simulink model "SolarInverter_DigitalTwin"  (R2019b)
settings: Solver=ode23tb  StartTime=0.0  StopTime=inf  RelTol=1e-3
InitFcn:
  | SolarInverter_Params();
values from neighbouring files (symbols this model uses):
  Fnom = 60    [SolarInverter_Params.m]
  Pnom = 112e3    (= 112000)    [SolarInverter_Params.m]
  reec_dbd1 = -0.1    [SolarInverter_Params.m]
  reec_dbd2 = 0.1    [SolarInverter_Params.m]
  reec_dPmax = 0.1    [SolarInverter_Params.m]
  reec_dPmin = -0.1    [SolarInverter_Params.m]
  reec_Imax = 1    [SolarInverter_Params.m]
  reec_Iqhl = 1.0    (= 1)    [SolarInverter_Params.m]
  reec_Iqll = -0.4    [SolarInverter_Params.m]
  reec_Kqi = 0.0    (= 0)    [SolarInverter_Params.m]
  reec_Kqp = 0    [SolarInverter_Params.m]
  reec_Kvi = 0.0    (= 0)    [SolarInverter_Params.m]
  reec_Kvp = 0.1    [SolarInverter_Params.m]
  reec_Pmax = 1.0    (= 1)    [SolarInverter_Params.m]
  reec_Pmin = 0    [SolarInverter_Params.m]
  reec_Qmax = 0.435    [SolarInverter_Params.m]
  reec_Qmin = -0.435    [SolarInverter_Params.m]
  reec_Tiq = 0.02    [SolarInverter_Params.m]
  reec_Tp = 0.02    [SolarInverter_Params.m]
  reec_Tpord = 0.1    [SolarInverter_Params.m]
  reec_Trv = 0.01    [SolarInverter_Params.m]
  reec_Vdip = 0.9    [SolarInverter_Params.m]
  reec_Vmax = 1.10    (= 1.1)    [SolarInverter_Params.m]
  reec_Vmin = 0.9    [SolarInverter_Params.m]
  reec_Vup = 1.15    [SolarInverter_Params.m]
  regc_Brkpt = 0.9    [SolarInverter_Params.m]
  regc_Iolim = -1.2    [SolarInverter_Params.m]
  regc_Iqrmax = 999.9    [SolarInverter_Params.m]
  regc_Iqrmin = -999.9    [SolarInverter_Params.m]
  regc_Ivpnt0 = 0.4    [SolarInverter_Params.m]
  regc_Ivpnt1 = 0.8    [SolarInverter_Params.m]
  regc_Khv = 0.0    (= 0)    [SolarInverter_Params.m]
  regc_Lvpl1 = 1.0    (= 1)    [SolarInverter_Params.m]
  regc_Lvplsw = 0    [SolarInverter_Params.m]
  regc_rrpwr = 10    [SolarInverter_Params.m]
  regc_Tfltr = 0.02    [SolarInverter_Params.m]
  regc_Tg = 0.1    [SolarInverter_Params.m]
  regc_Volim = 1.1    [SolarInverter_Params.m]
  regc_Zerox = 0.5    [SolarInverter_Params.m]
  repc_db1 = 0    [SolarInverter_Params.m]
  repc_Ddn = 20    [SolarInverter_Params.m]
  repc_Dup = 0    [SolarInverter_Params.m]
  repc_emax = 999    [SolarInverter_Params.m]
  repc_emin = -999    [SolarInverter_Params.m]
  repc_fdbd1 = 0.01*0    (= 0)    [SolarInverter_Params.m]
  repc_fdbd2 = -0.01*0    (= 0)    [SolarInverter_Params.m]
  repc_femax = 999    [SolarInverter_Params.m]
  repc_femin = -999    [SolarInverter_Params.m]
  repc_Kc = 0.05    [SolarInverter_Params.m]
  repc_Ki = 1.8    [SolarInverter_Params.m]
  repc_Kig = 0.5    [SolarInverter_Params.m]
  repc_Kp = 0.6    [SolarInverter_Params.m]
  repc_Kpg = 0.1    [SolarInverter_Params.m]
  repc_Pmax = 1    [SolarInverter_Params.m]
  repc_Pmin = 0    [SolarInverter_Params.m]
  repc_Qmax = inf    [SolarInverter_Params.m]
  repc_Qmin = -inf    [SolarInverter_Params.m]
  repc_Rc = 0    [SolarInverter_Params.m]
  repc_Tfltr = 0.02    [SolarInverter_Params.m]
  repc_Tft = 0.5    [SolarInverter_Params.m]
  repc_Tfv = 0.8    [SolarInverter_Params.m]
  repc_Tlag = 0.2    [SolarInverter_Params.m]
  repc_Tp = 0.25    [SolarInverter_Params.m]
  repc_Vfrz = 0.7    [SolarInverter_Params.m]
  repc_Xc = 0    [SolarInverter_Params.m]
  Vnom = 142e3    (= 142000)    [SolarInverter_Params.m]
undefined symbols (not defined in the file or in its folder): gcbh, j, sps_rtmsupport
libraries: simulink x15, powerlib x7, powerlib_meascontrol x2
(part 1 of 2)
settings Model: EnablePacing=on  OrderedModelArguments=off  Creator=jlesage  LastModifiedBy=jlesage
settings SolverCC: ZeroCrossAlgorithm=Adaptive
settings DataIOCC: InitialState=getstatestruct(opreport)  SaveOutput=off  SignalLogging=off  DSMLogging=off  SaveTime=off  ReturnWorkspaceOutputs=off
settings DebuggingCC: IgnoredZcDiagnostic=none
settings SFSimCC: CustomCodeUndefinedFunction=UseInterfaceOnly

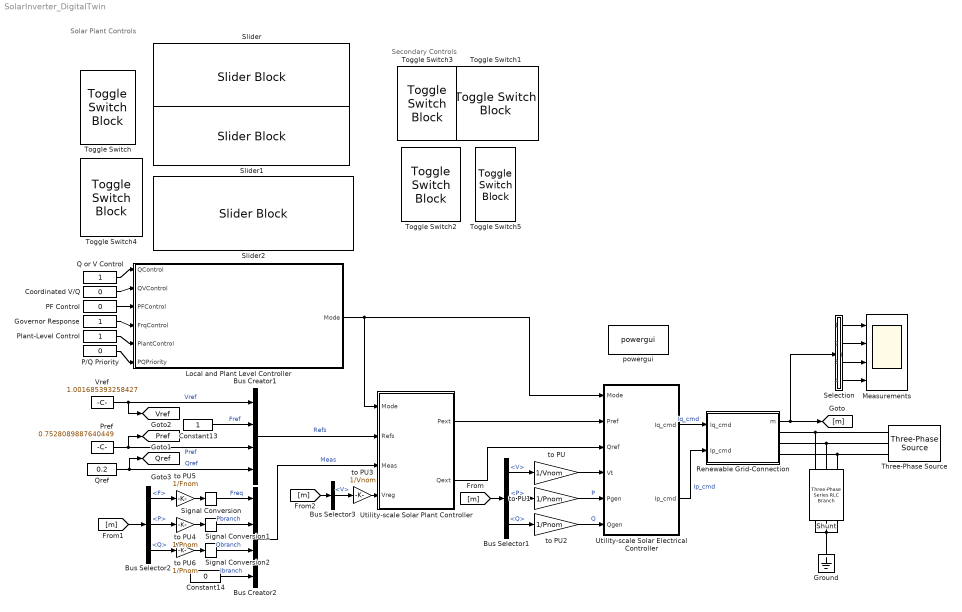
== system SolarInverter_DigitalTwin ==
  note: Solar Plant Controls
  note: Secondary Controls
  Bus Creator1 : BusCreator  Inputs=4
  Bus Creator2 : BusCreator  Inputs=4
  Bus Selector1 : BusSelector  OutputSignals=V,P,Q
  Bus Selector2 : BusSelector  OutputSignals=F,P,Q
  Bus Selector3 : BusSelector  OutputSignals=V
  Constant13 : Constant
  Constant14 : Constant  Value=0
  Coordinated V/Q : Constant  Value=0
  Governor Response : Constant
  Ground : powerlib/Elements/Ground  LConnTagsString=a
      settings: SourceProductName=Simscape Electrical
  Local and Plant Level Controller : Stateflow chart  InitFcn=|  BlockKeywords=__PRM__SERIALIZED__DATA__:Stateflow Chart,Stateflow Diagram  TreatAsAtomicUnit=on
      | BusElement(1) = Simulink.BusElement;
      | BusElement(1).Name = 'QFlag';
      | BusElement(1).Dimensions = 1;
      | BusElement(1).DimensionsMode = 'Fixed';
      | BusElement(1).DataType = 'double';
      | BusElement(1).Complexity = 'real';
      | 
      | BusElement(2) = Simulink.BusElement;
      | BusElement(2).Name = 'VFlag';
      | BusElement(2).Dimensions = 1;
      | BusElement(2).DimensionsMode = 'Fixed';
      | BusElement(2).DataType = 'double';
      | BusElement(2).Complexity = 'real';
      | 
      | BusElement(3) = Simulink.BusElement;
      | BusElement(3).Name = 'PfFlag';
      | BusElement(3).Dimensions = 1;
      | BusElement(3).DimensionsMode = 'Fixed';
      | BusElement(3).DataType = 'double';
      | BusElement(3).Complexity = 'real';
      | 
      | BusElement(4) = Simulink.BusElement;
      | BusElement(4).Name = 'PqFlag';
      | BusElement(4).Dimensions = 1;
      | BusElement(4).DimensionsMode = 'Fixed';
      | BusElement(4).DataType = 'double';
      | BusElement(4).Complexity = 'real';
      | 
      | BusElement(5) = Simulink.BusElement;
      | BusElement(5).Name = 'VcompFlag';
      | BusElement(5).Dimensions = 1;
      | BusElement(5).DimensionsMode = 'Fixed';
      | BusElement(5).DataType = 'double';
      | BusElement(5).Complexity = 'real';
      | 
      | BusElement(6) = Simulink.BusElement;
      | BusElement(6).Name = 'RefFlag';
      | BusElement(6).Dimensions = 1;
      | BusElement(6).DimensionsMode = 'Fixed';
      | BusElement(6).DataType = 'double';
      | BusElement(6).Complexity = 'real';
      | 
      | BusElement(7) = Simulink.BusElement;
      | BusElement(7).Name = 'FrqFlag';
      | BusElement(7).Dimensions = 1;
      | BusElement(7).DimensionsMode = 'Fixed';
      | BusElement(7).DataType = 'double';
      | BusElement(7).Complexity = 'real';
      | 
      | Mode = Simulink.Bus;
      | Mode.Elements = BusElement;
      | 
      | clearvars BusElement
  Measurements : Scope  NumInputPorts=4
  P/Q Priority : Constant  Value=0
  PF Control : Constant  Value=0
  Plant-Level Control : Constant
  Pref : Constant  Value=0.7528089887640449
  Q or V Control : Constant
  Qref : Constant  Value=0.2
  Renewable Grid-Connection : Subsystem  mask(Renewable Energy Grid Connection (REGC_A)){Tfltr=regc_Tfltr, Lvpl1=regc_Lvpl1, Zerox=regc_Zerox, Brkpt=regc_Brkpt, Lvplsw=regc_Lvplsw, rrpwr=regc_rrpwr, Tg=regc_Tg, Volim=regc_Volim, Iolim=regc_Iolim, Khv=regc_Khv, Ivpnt0=regc_Ivpnt0, Ivpnt1=regc_Ivpnt1, Iqrmax=regc_Iqrmax, Iqrmin=regc_Iqrmin}
      mask prompts: Tfltr "Tfltr - Terminal Voltage Filter [s]"; Lvpl1 "Lvpl1 - LVPL Gain Breakpoint [pu]"; Zerox "Zerox - LVPL Zero Crossing [pu]"; Brkpt "Brkpt - LVPL Breakpoint [pu]"; Lvplsw "Lvplsw - Low Voltage Power Logic [Enable (1) or Disable (0)]"; rrpwr "rrpwr - Active Current up-ramp rater limit [pu/s]"; Tg "Tg - Inverter Current Lag Time [s]"; Volim "Volim - Voltage Limit Clap Logic [pu]"; Iolim "Iolim - Current Limit for Clap Logic [pu]"; Khv "Khv - High Voltage Clap Logic Factor"; Ivpnt0 "Ivpnt0 - Low voltage current breakpoint [pu]"; Ivpnt1 "Ivpnt1 - Low voltage current breakpoint [pu]"; Iqrmax "Iqrmax - Maximum rate of change [pu/s]"; Iqrmin "Iqrmin - Minimum rate of change [pu/s]"
      mask help: REGC_A module, used to represent the Generator/Converter (inverter) interface with the grid. It processes the real and reactive current command and outputs of real and reactive current injection into the grid model.
      mask Display: color('blue');disp('REGC_A')
  Selection : Subsystem
  Shunt : powerlib/Elements/Three-Phase Series RLC Branch  LConnTagsString=A|B|C  RConnTagsString=A|B|C  BranchType=R  Resistance=1e9  Inductance=0  Capacitance=1e-6  Measurements=None
      settings: SourceProductName=Simscape Electrical
  Signal Conversion : SignalConversion  OverrideOpt=off
  Signal Conversion1 : SignalConversion  OverrideOpt=off
  Signal Conversion2 : SignalConversion  OverrideOpt=off
  Slider : SliderBlock  ScaleMin=0.94999999999999996  ScaleMax=1.05
  Slider1 : SliderBlock  ScaleMax=1  TickInterval=0.25
  Slider2 : SliderBlock  ScaleMin=-1  ScaleMax=1
  Three-Phase Source : powerlib/Electrical Sources/Three-Phase Source  InternalConnection=Yg  VoltagePhases=off  Voltage=Vnom*0.995  PhaseAngle=0  Voltage_phases=[25e3 25e3 25e3]/sqrt(3)  PhaseAngles_phases=[0 -120 +120]  Frequency=60  NonIdealSource=on  SpecifyImpedance=on  Resistance=0.8929  Inductance=16.58e-3  ShortCircuitLevel=20e5  BaseVoltage=Vnom  XRratio=10  BusType=swing  Pref=10e3  Qref=0  Prefabc=[10e3, 10e3, 10e3]  Qrefabc=[0, 0, 0]  Qmin=-inf  Qmax=inf
      settings: SourceProductName=Simscape Electrical
  Toggle Switch{,1..5} (6 alike) : ToggleSwitchBlock  LabelPosition=Hide
  Utility-scale Solar Electrical Controller : Subsystem  mask(Renewable Energy Electrical Controller (REEC_B)){Trv=reec_Trv, Vdip=reec_Vdip, Vup=reec_Vup, dbd1=reec_dbd1, dbd2=reec_dbd2, Kqv=0, Iqhl=reec_Iqhl, Iqll=reec_Iqll, Tp=reec_Tp, Qmax=reec_Qmax, Qmin=reec_Qmin, Kqp=reec_Kqp, Kqi=reec_Kqi, Vmax=reec_Vmax, Vmin=reec_Vmin, Kvp=reec_Kvp, Kvi=reec_Kvi, Tiq=reec_Tiq, Tpord=reec_Tpord, Pmax=reec_Pmax, Pmin=reec_Pmin, dPmax=reec_dPmax, dPmin=reec_dPmin, Imax=reec_Imax}
      mask prompts: Trv "Trv - Terminal Bus Filter [s]"; Vdip "Vdip - Low Voltage Trigger [pu]"; Vup "Vup - High Voltage Trigger [pu]"; dbd1 "dbd1 - Overvoltage deadband [pu]"; dbd2 "dbd2 - Undervoltage deadband [pu]"; Kqv "Kqv - Reactive current injection gain [pu]"; Iqhl "Iqhl - Maximum current injection [pu]"; Iqll "Iqll - Minimum current injection [pu]"; Tp "Tp - Active Power Time Constant [s]"; Qmax "Qmax - Maximum reactive power [pu]"; Qmin "Qmin - Minimum reactive power [pu]"; Kqp "Kqp - Local Q regulator [pu]"; Kqi "Kqi - Local Q integrator gain [pu]"; Vmax "Vmax - Maximum inverter voltage [pu]"; Vmin "Vmin - Minium inverter terminal voltage [pu]"; Kvp "Kvp - Voltage Regulator Gain [pu]"; Kvi "Kvi - Voltage Integrator Gain [pu]"; Tiq "Tiq - Reactive Power Lag [s]"; Tpord "Tpord - Inverter Lag Time Constant [s]"; Pmax "Pmax - Maximum active power [pu]"; Pmin "Pmin - Minimum active power [pu]"; dPmax "dPmax - Power Up-ramp Limit [pu/s]"; dPmin "dPmin - Power Down-ramp Limit [pu/s]"; Imax "Imax - Maximum apparent current [pu]"
      mask help: REEC_B module, used to represent the Electrical Controls of the inverters. It acts on the active and reactive power reference from the REPC_A module, with feedback of terminal voltage and generator power output, and provides real and reactive current commands to the REGC_A module.
      mask Display: color('blue');disp('REEC_A')
  Utility-scale Solar Plant Controller : Subsystem  mask(Renewable Energy Plant Controller (REPC_A)){Tfltr=repc_Tfltr, Xc=repc_Xc, Rc=repc_Rc, Kc=repc_Kc, db1=repc_db1, emax=repc_emax, emin=repc_emin, Kp=repc_Kp, Ki=repc_Ki, Qmax=repc_Qmax, Qmin=repc_Qmin, Vfrz=repc_Vfrz, Tft=repc_Tft, Tfv=repc_Tfv, fdbd1=repc_fdbd1, fdbd2=repc_fdbd2, Ddn=repc_Ddn, Dup=repc_Dup, Tp=repc_Tp, femax=repc_femax, femin=repc_femin, Kpg=repc_Kpg, Kig=repc_Kig, Tlag=repc_Tlag, Pmax=repc_Pmax, Pmin=repc_Pmin}
      mask prompts: Tfltr "Tfltr - Voltage/Reactive Power Time Constants [s]"; Xc "Xc - Line drop compensation reactance [pu]"; Rc "Rc - Line drop compensation resistance [pu]"; Kc "Kc - Reactive droop [pu]"; db1 "db - Reactive power deadline [pu]"; emax "emax - Maximum Volt/VAR error [pu]"; emin "emin - Minimum Volt/VAR error [pu]"; Kp "Kp - Volt/VAR Propotional Gain [pu/pu]"; Ki "Ki - Volt/VAR Integral Gain [pu/pu-s]"; Qmax "Qmax - Max Plant Reactive Power [pu]"; Qmin "Qmin - Min Plant Reactive Power [pu]"; Vfrz "Vfrz - Voltage for Freezing Volt/VAR Integrator [pu]"; Tft "Tft - Q Lead Time Constant [s]"; Tfv "Tfv - Q Lag Time Constant [s]"; fdbd1 "fdbd1 - Overfrequency deadband for govenor [pu]"; fdbd2 "fdbd2 - Underfrequency deadband for govenor [pu]"; Ddn "Ddn - Down regulation droop [pu]"; Dup "Dup - Up regulation droop [pu]"; Tp "Tp - Active Power Filter Time Constant [s]"; femax "femax - Maximum Power Error [pu]"; femin "femin - Minimum Power Error [pu]"; Kpg "Kpg - Droop regulator gain [pu]"; Kig "Kig - Droop integral gain [pu]"; Tlag "Tlag - Plant Controller P output Lag [s]"; Pmax "Pmax - Maximum Plant Active Power [pu]"; Pmin "Pmin - Minimum Plant Active Power [pu]"
      mask help: REPC_A module, used to represent the Plant Controller. It processes voltage and reactive power output to emulate volt/var control at the plant level. It also processes frequency and active power output to emulate active power control. This module provides active reactive power command to the REEC_B module.
      mask Display: color('blue');disp('REPC_A')
  Vref : Constant  Value=1.001685393258427
  powergui : powerlib/powergui  Priority=1  SimulationMode=Phasor  SampleTime=50e-6  frequency=60  Iterations=50  frequencyindice=60  Pbase=100e6  ErrMax=1e-4  UnitsV=kV  UnitsW=MW  buscounter=0  FunctionMessages=off  echomessages=off  EnableUseOfTLC=off  CurrentSourceSwitches=off  DisableSnubberDevices=off  DisableRonSwitches=off  DisableVfSwitches=off  DisplayEquations=off  AutomaticDiscreteSolvers=off  SolverType=Tustin/Backward Euler (TBE)  Interpol=off  ExternalGateDelay=off  methode=off  Ts=100  x0status=blocks  SPID=on  SwTol=0  HookPort=off  NonlinearTolerance=0  nMaxIteration=15  ContinueOnMaxIteration=off  RestoreLinks=warning  ResistiveCurrentMeasurement=off  Frange=[0:2:500]  Ylog=off  Xlog=on  ShowGrid=off  save=off  variable=ZData  structure=0  ZoomFFT=off  StartTime=0.0  cycles=1  DisplayStyle=1  fundamental=60  FreqAxis=off  MaxFrequency=1000  frequencyindicesteady=1  RmsSteady=1  display=off
      settings: SourceProductName=Simscape Electrical
  to PU : Gain  Gain=1/Vnom
  to PU{1..2,4,6} (4 alike) : Gain  Gain=1/Pnom
  to PU3 : Gain  Gain=1/Vnom
  to PU5 : Gain  Gain=1/Fnom
  tag scope: Pref=global, Qref=global, Vref=global
  wires:
  Renewable Grid-Connection/1(m) -> [m], Selection/1(In1)
  Utility-scale Solar Plant Controller/1(Pext) -> Utility-scale Solar Electrical Controller/2(Pref)
  Bus Selector1/3 -> to PU2/1  "<Q>"
  Bus Selector1/1 -> to PU/1  "<V>"
  Bus Selector1/2 -> to PU1/1  "<P>"
  [m] -> Bus Selector1/1
  to PU/1 -> Utility-scale Solar Electrical Controller/4(Vt)
  Utility-scale Solar Electrical Controller/1(Iq_cmd) -> Renewable Grid-Connection/1(Iq_cmd)  "Iq_cmd"
  Utility-scale Solar Electrical Controller/2(Ip_cmd) -> Renewable Grid-Connection/2(Ip_cmd)  "Ip_cmd"
  to PU1/1 -> Utility-scale Solar Electrical Controller/5(Pgen)  "P"
  to PU2/1 -> Utility-scale Solar Electrical Controller/6(Qgen)  "Q"
  Bus Selector2/3 -> to PU6/1  "<Q>"
  to PU6/1 -> Signal Conversion2/1
  Signal Conversion2/1 -> Bus Creator2/3  "Qbranch"
  Signal Conversion/1 -> Bus Creator2/1  "Freq"
  to PU3/1 -> Utility-scale Solar Plant Controller/4(Vreg)
  Bus Creator1/1 -> Utility-scale Solar Plant Controller/2(Refs)  "Refs"
  Signal Conversion1/1 -> Bus Creator2/2  "Pbranch"
  to PU5/1 -> Signal Conversion/1
  Constant13/1 -> Bus Creator1/2  "Fref"
  Bus Selector2/2 -> to PU4/1  "<P>"
  [m] -> Bus Selector3/1
  Pref/1 -> Bus Creator1/3, [Pref]  "Pref"
  Bus Creator2/1 -> Utility-scale Solar Plant Controller/3(" Meas")  "Meas"
  Constant14/1 -> Bus Creator2/4  "Ibranch"
  Bus Selector2/1 -> to PU5/1  "<F>"
  Qref/1 -> [Qref], Bus Creator1/4  "Qref"
  [m] -> Bus Selector2/1
  to PU4/1 -> Signal Conversion1/1
  Bus Selector3/1 -> to PU3/1  "<V>"
  Utility-scale Solar Plant Controller/2(Qext) -> Utility-scale Solar Electrical Controller/3(Qref)
  Vref/1 -> Bus Creator1/1, [Vref]  "Vref"
  Local and Plant Level Controller/1(Mode) -> Utility-scale Solar Plant Controller/1(Mode), Utility-scale Solar Electrical Controller/1(Mode)
  P/Q Priority/1 -> Local and Plant Level Controller/6(PQPriority)
  Plant-Level Control/1 -> Local and Plant Level Controller/5(PlantControl)
  Governor Response/1 -> Local and Plant Level Controller/4(FrqControl)
  PF Control/1 -> Local and Plant Level Controller/3(PFControl)
  Coordinated V/Q/1 -> Local and Plant Level Controller/2(QVControl)
  Q or V Control/1 -> Local and Plant Level Controller/1(QControl)
  Selection/1(Out1) -> Measurements/1
  Selection/2(<F>) -> Measurements/2
  Selection/3(Out3) -> Measurements/3
  Selection/4(Out4) -> Measurements/4
  connections:
  Shunt/LConn3 -- Three-Phase Source/RConn3 -- Renewable Grid-Connection/RConn3
  Shunt/LConn1 -- Three-Phase Source/RConn1 -- Renewable Grid-Connection/RConn1
  Shunt/RConn2 -- Ground/LConn1 -- Shunt/RConn3 -- Shunt/RConn1
  Shunt/LConn2 -- Three-Phase Source/RConn2 -- Renewable Grid-Connection/RConn2

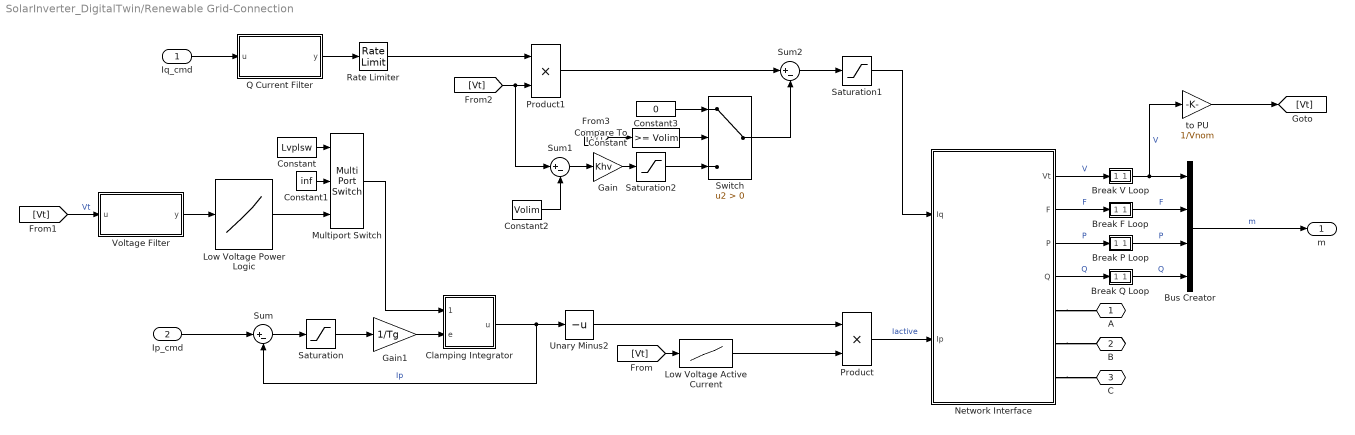
== system SolarInverter_DigitalTwin/Renewable Grid-Connection ==
  Iq_cmd : Inport
  Ip_cmd : Inport  Port=2
  Break F Loop : Subsystem  mask{tau=0.001, toPU=Fnom}
      mask prompts: toPU "Convert to PU"
  Break P Loop : Subsystem  mask{tau=0.001, toPU=Pnom}
      mask prompts: toPU "Convert to PU"
  Break Q Loop : Subsystem  mask{tau=0.001, toPU=Pnom}
      mask prompts: toPU "Convert to PU"
  Break V Loop : Subsystem  mask{tau=0.001, toPU=Vnom}
      mask prompts: toPU "Convert to PU"
  Bus Creator : BusCreator  Inputs=4
  Clamping Integrator : Subsystem
  Compare To Constant : simulink/Logic and Bit Operations/Compare To Constant  relop=>=  const=Volim  OutDataTypeStr=boolean
  Constant : Constant  Value=Lvplsw
  Constant1 : Constant  Value=inf
  Constant2 : Constant  Value=Volim
  Constant3 : Constant  Value=0
  Gain : Gain  Gain=Khv
  Gain1 : Gain  Gain=1/Tg
  Low Voltage Active Current : Lookup_n-D  NumberOfTableDimensions=1  BreakpointsForDimension1=[0 Ivpnt0 Ivpnt1 Ivpnt1*1.5]  Table=[0 0 1 1]  InternalRulePriority=Speed  RndMeth=Simplest  InputSameDT=on
  Low Voltage Power Logic : Lookup_n-D  NumberOfTableDimensions=1  BreakpointsForDimension1=[0 Zerox Brkpt Brkpt*1.01 Brkpt*1.5]  Table=[0 0 Lvpl1 Lvpl1*5 Lvpl1*5]  InternalRulePriority=Speed  RndMeth=Simplest  InputSameDT=on
  Multiport Switch : MultiPortSwitch  DataPortOrder=Zero-based contiguous  Inputs=2  zeroidx=on
  Network Interface : Subsystem
  Product : Product
  Product1 : Product
  Q Current Filter : Subsystem  mask{k=1, tau=Tg, vmax=Iqrmax, vmin=Iqrmin}
      mask Display: fprintf('1\n------------\n(1 + s Tg)');
  Rate Limiter : RateLimiter  RisingSlewLimit=Iqrmax  FallingSlewLimit=Iqrmin  SampleTimeMode=inherited
  Saturation : Saturate  UpperLimit=rrpwr  LowerLimit=-inf
  Saturation1 : Saturate  UpperLimit=inf  LowerLimit=Iolim
  Saturation2 : Saturate  UpperLimit=inf  LowerLimit=0
  Sum : Sum  Inputs=|+-
  Sum1 : Sum  Inputs=|+-
  Sum2 : Sum  Inputs=|+-
  Switch : Switch  Criteria=u2 > Threshold
  Unary Minus2 : UnaryMinus
  Voltage Filter : Subsystem  mask{k=1, tau=Tfltr, vmax=inf, vmin=-inf}
      mask Display: fprintf('1\n------------\n(1 + s Tfltr)');
  to PU : Gain  Gain=1/Vnom
  A : PMIOPort  Side=Right
  B : PMIOPort  Port=2  Side=Right
  C : PMIOPort  Port=3  Side=Right
  m : Outport  VectorParamsAs1DForOutWhenUnconnected=off
  wires:
  [Vt] -> Voltage Filter/1(u)  "Vt"
  Q Current Filter/1(y) -> Rate Limiter/1
  Network Interface/4(Q) -> Break Q Loop/1(u)  "Q"
  Constant3/1 -> Switch/1
  Network Interface/1(Vt) -> Break V Loop/1(u)  "V"
  Iq_cmd/1 -> Q Current Filter/1(u)
  Gain/1 -> Saturation2/1
  Network Interface/3(P) -> Break P Loop/1(u)  "P"
  Voltage Filter/1(y) -> Low Voltage Power Logic/1
  Constant1/1 -> Multiport Switch/2
  Sum/1 -> Saturation/1
  Constant/1 -> Multiport Switch/1
  Product/1 -> Network Interface/2(Ip)  "Iactive"
  Low Voltage Active Current/1 -> Product/2
  Multiport Switch/1 -> Clamping Integrator/1(LVMax)
  Clamping Integrator/1(u) -> Sum/2, Unary Minus2/1  "Ip"
  Gain1/1 -> Clamping Integrator/2(e)
  [Vt] -> Compare To Constant/1
  Saturation/1 -> Gain1/1
  [Vt] -> Low Voltage Active Current/1
  Constant2/1 -> Sum1/2
  Saturation1/1 -> Network Interface/1(Iq)
  Product1/1 -> Sum2/1
  Sum1/1 -> Gain/1
  Rate Limiter/1 -> Product1/1
  Saturation2/1 -> Switch/3
  [Vt] -> Sum1/1, Product1/2
  Low Voltage Power Logic/1 -> Multiport Switch/3
  Compare To Constant/1 -> Switch/2
  Switch/1 -> Sum2/2
  Bus Creator/1 -> m/1  "m"
  Sum2/1 -> Saturation1/1
  Ip_cmd/1 -> Sum/1
  Network Interface/2(F) -> Break F Loop/1(u)  "F"
  Unary Minus2/1 -> Product/1
  to PU/1 -> [Vt]
  Break V Loop/1(y) -> to PU/1, Bus Creator/1  "V"
  Break F Loop/1(y) -> Bus Creator/2  "F"
  Break P Loop/1(y) -> Bus Creator/3  "P"
  Break Q Loop/1(y) -> Bus Creator/4  "Q"
  connections:
  Network Interface/RConn3 -- C/RConn1
  Network Interface/RConn1 -- A/RConn1
  Network Interface/RConn2 -- B/RConn1

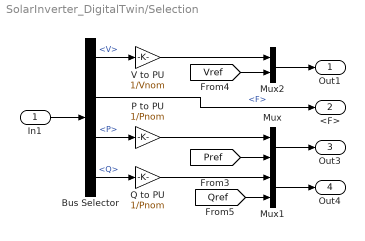
== system SolarInverter_DigitalTwin/Selection ==
  In1 : Inport
  Bus Selector : BusSelector  OutputSignals=V,F,P,Q
  Mux : Mux  Inputs=2
  Mux1 : Mux  Inputs=2
  Mux2 : Mux  Inputs=2
  P to PU : Gain  Gain=1/Pnom
  Q to PU : Gain  Gain=1/Pnom
  V to PU : Gain  Gain=1/Vnom
  Out1 : Outport
  <F> : Outport  Port=2
  Out3 : Outport  Port=3
  Out4 : Outport  Port=4
  wires:
  Bus Selector/4 -> Q to PU/1  "<Q>"
  Bus Selector/3 -> P to PU/1  "<P>"
  V to PU/1 -> Mux2/1
  Bus Selector/1 -> V to PU/1  "<V>"
  [Vref] -> Mux2/2
  Q to PU/1 -> Mux1/1
  P to PU/1 -> Mux/1
  [Qref] -> Mux1/2
  [Pref] -> Mux/2
  Bus Selector/2 -> <F>/1  "<F>"
  Mux/1 -> Out3/1
  Mux2/1 -> Out1/1
  Mux1/1 -> Out4/1
  In1/1 -> Bus Selector/1

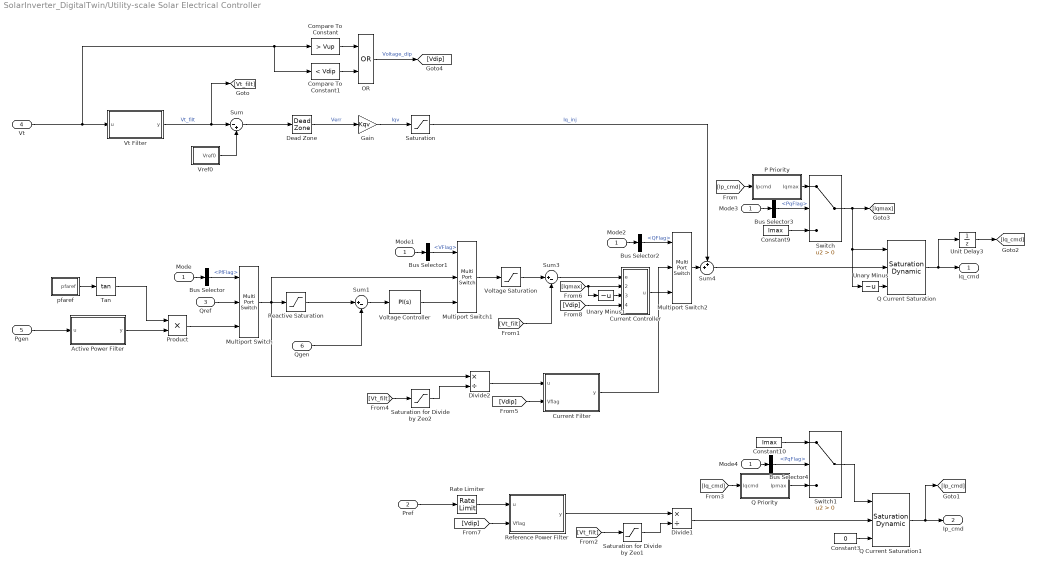
== system SolarInverter_DigitalTwin/Utility-scale Solar Electrical Controller ==
  Mode : Inport
  Pref : Inport  Port=2
  Qref : Inport  Port=3
  Vt : Inport  Port=4
  Pgen : Inport  Port=5
  Qgen : Inport  Port=6
  Active Power Filter : Subsystem  mask{k=1, tau=Tp, vmax=Inf, vmin=-Inf}
      mask Display: fprintf('1\n------------\n(1 + s Tp)');
  Bus Selector : BusSelector  OutputSignals=PfFlag
  Bus Selector1 : BusSelector  OutputSignals=VFlag
  Bus Selector2 : BusSelector  OutputSignals=QFlag
  Bus Selector3 : BusSelector  OutputSignals=PqFlag
  Bus Selector4 : BusSelector  OutputSignals=PqFlag
  Compare To Constant : simulink/Logic and Bit Operations/Compare To Constant  relop=>  const=Vup  OutDataTypeStr=boolean
  Compare To Constant1 : simulink/Logic and Bit Operations/Compare To Constant  relop=<  const=Vdip  OutDataTypeStr=boolean
  Constant10 : Constant  Value=Imax
  Constant3 : Constant  Value=0
  Constant9 : Constant  Value=Imax
  Current Controller : Subsystem
  Current Filter : Subsystem  mask{k=1, tau=Tiq, vmax=Inf, vmin=-Inf}
      mask Display: fprintf('1\n------------\n(1 + s Tiq)');
  Dead Zone : DeadZone  LowerValue=dbd1  UpperValue=dbd2  SaturateOnIntegerOverflow=on
  Divide1 : Product  Inputs=*/
  Divide2 : Product  Inputs=*/
  Gain : Gain  Gain=Kqv
  Mode{1..4} (4 alike) : InportShadow
  Multiport Switch : MultiPortSwitch  DataPortOrder=Zero-based contiguous  Inputs=2  zeroidx=on
  Multiport Switch1 : MultiPortSwitch  DataPortOrder=Zero-based contiguous  Inputs=2  zeroidx=on
  Multiport Switch2 : MultiPortSwitch  DataPortOrder=Zero-based contiguous  Inputs=2  zeroidx=on
  OR : Logic  Operator=OR  AllPortsSameDT=off  OutDataTypeStr=boolean
  P Priority : Subsystem
  Product : Product
  Q Current Saturation : simulink/Discontinuities/Saturation Dynamic  OutMin=[]  OutMax=[]  OutDataTypeStr=Inherit: Same as second input  OutDataType=fixdt(1, 16)  OutScaling=2^-10  DoSatur=off
  Q Current Saturation1 : simulink/Discontinuities/Saturation Dynamic  OutMin=[]  OutMax=[]  OutDataTypeStr=Inherit: Same as second input  OutDataType=fixdt(1, 16)  OutScaling=2^-10  DoSatur=off
  Q Priority : Subsystem
  Rate Limiter : RateLimiter  RisingSlewLimit=dPmax  FallingSlewLimit=dPmin  SampleTimeMode=inherited
  Reactive Saturation : Saturate  UpperLimit=Qmax  LowerLimit=Qmin
  Reference Power Filter : Subsystem  mask{k=1, tau=Tpord, vmax=Pmax, vmin=Pmin}
      mask Display: fprintf('1\n------------\n(1 + s Tpord)');
  Saturation : Saturate  UpperLimit=Iqhl  LowerLimit=Iqll
  Saturation for Divide by Zeo1 : Saturate  UpperLimit=inf  LowerLimit=0.01
  Saturation for Divide by Zeo2 : Saturate  UpperLimit=inf  LowerLimit=0.01
  Sum : Sum  Inputs=|-+
  Sum1 : Sum  Inputs=|+-
  Sum3 : Sum  Inputs=|+-
  Sum4 : Sum  Inputs=++|
  Switch : Switch  Criteria=u2 > Threshold
  Switch1 : Switch  Criteria=u2 > Threshold
  Tan : Trigonometry  Operator=tan
  Unary Minus : UnaryMinus
  Unary Minus1 : UnaryMinus
  Unit Delay3 : UnitDelay  SampleTime=-1  HasFrameUpgradeWarning=on
  Voltage Controller : simulink/Continuous/PID Controller  Controller=PI  Form=Parallel  TimeDomain=Continuous-time  SampleTime=-1  IntegratorMethod=Forward Euler  FilterMethod=Forward Euler  ControllerParametersSource=internal  P=Kqp  I=Kqi  D=0  UseFilter=on  N=100  TunerSelectOption=Transfer Function Based (PID Tuner App)  InitialConditionSource=internal  InitialConditionForIntegrator=1  InitialConditionForFilter=0  DifferentiatorICPrevScaledInput=0  ExternalReset=none  TrackingMode=off  Kt=1  LimitOutput=on  UpperSaturationLimit=Vmax  LowerSaturationLimit=Vmin  LinearizeAsGain=on  AntiWindupMode=none  Kb=1  POutMin=[]  POutMax=[]  IOutMin=[]  IOutMax=[]  DOutMin=[]  DOutMax=[]  NOutMin=[]  NOutMax=[]  SumOutMin=[]  SumOutMax=[]  SaturationOutMin=[]  SaturationOutMax=[]  PParamMin=[]  PParamMax=[]  IParamMin=[]  IParamMax=[]  DParamMin=[]  DParamMax=[]  NParamMin=[]  NParamMax=[]  KbParamMin=[]  KbParamMax=[]  KtParamMin=[]  KtParamMax=[]  KbOutMin=[]  KbOutMax=[]  KtOutMin=[]  KtOutMax=[]  IntegratorOutMin=[]  IntegratorOutMax=[]  FilterOutMin=[]  FilterOutMax=[]  SumI1OutMin=[]  SumI1OutMax=[]  SumI2OutMin=[]  SumI2OutMax=[]  SumI3OutMin=[]  SumI3OutMax=[]  SumI4OutMin=[]  SumI4OutMax=[]  SumDOutMin=[]  SumDOutMax=[]  DifferentiatorOutMin=[]  DifferentiatorOutMax=[]  FilterDiffOutCoefMin=[]  FilterDiffOutCoefMax=[]  ReciprocalOutMin=[]  ReciprocalOutMax=[]  SumDenOutMin=[]  SumDenOutMax=[]  SumNumOutMin=[]  SumNumOutMax=[]  DivideOutMin=[]  DivideOutMax=[]  IntegratorContinuousStateAttributes=''  IntegratorStateMustResolveToSignalObject=off  IntegratorRTWStateStorageClass=Auto  FilterContinuousStateAttributes=''  FilterStateMustResolveToSignalObject=off  FilterRTWStateStorageClass=Auto  ParallelPVariant=InternalParameters  IdealPVariant=Disabled  IVariant=InternalParameters  DVariant=Disabled  IntegratorVariant=Continuous  SatVariant=Enabled  AWVariant=Passthrough  PCopyVariant=Disabled  TRVariant=Disabled  FdbkBlocksVariant=Forward  IdealPFdbkVariant=Disabled  SatFdbkVariant=Disabled  DerivativeFilterVariant=Disabled  NVariant=Disabled  NCopyVariant=Disabled_SignalSpec  FilterICVariant=Disabled  IntegratorICVariant=InternalICs  ExternalResetVariant=Disabled  TRSumVariant=Passthrough  SumFdbkVariant=Disabled  SumVariant=Sum_PI
  Voltage Saturation : Saturate  UpperLimit=Vmax  LowerLimit=Vmin
  Vref0 : Subsystem
  Vt Filter : Subsystem  mask{k=1, tau=Trv, vmax=Inf, vmin=-Inf}
      mask Display: fprintf('1\n------------\n(1 + s Trv)');
  pfaref : Subsystem
  Iq_cmd : Outport  VectorParamsAs1DForOutWhenUnconnected=off
  Ip_cmd : Outport  Port=2  VectorParamsAs1DForOutWhenUnconnected=off
  wires:
  Unit Delay3/1 -> [Iq_cmd]
  Qgen/1 -> Sum1/2
  Pgen/1 -> Active Power Filter/1(u)
  Vt/1 -> Vt Filter/1(u), Compare To Constant/1, Compare To Constant1/1
  Vref0/1(Vref0) -> Sum/2
  Reactive Saturation/1 -> Sum1/1
  Voltage Controller/1 -> Multiport Switch1/3
  Bus Selector4/1 -> Switch1/2  "<PqFlag>"
  Sum/1 -> Dead Zone/1
  Multiport Switch/1 -> Reactive Saturation/1, Multiport Switch1/2, Divide2/1
  Voltage Saturation/1 -> Sum3/1
  Bus Selector2/1 -> Multiport Switch2/1  "<QFlag>"
  Vt Filter/1(y) -> Sum/1, [Vt_filt]  "Vt_filt"
  [Iqmax] -> Current Controller/2(umax), Unary Minus1/1
  Constant10/1 -> Switch1/1
  [Vt_filt] -> Sum3/2
  Dead Zone/1 -> Gain/1  "Verr"
  Tan/1 -> Product/1
  Sum3/1 -> Current Controller/1(e)
  Product/1 -> Multiport Switch/3
  Current Controller/1(u) -> Multiport Switch2/3
  Rate Limiter/1 -> Reference Power Filter/1(u)
  Q Current Saturation/1 -> Unit Delay3/1, Iq_cmd/1
  [Vt_filt] -> Saturation for Divide by Zeo1/1
  Current Filter/1(y) -> Multiport Switch2/2
  Sum4/1 -> Q Current Saturation/2
  Unary Minus/1 -> Q Current Saturation/3
  Multiport Switch2/1 -> Sum4/2
  Saturation for Divide by Zeo2/1 -> Divide2/2
  Pref/1 -> Rate Limiter/1
  Multiport Switch1/1 -> Voltage Saturation/1
  Divide1/1 -> Q Current Saturation1/2
  Divide2/1 -> Current Filter/1(u)
  Saturation for Divide by Zeo1/1 -> Divide1/2
  [Ip_cmd] -> P Priority/1(Ipcmd)
  Reference Power Filter/1(y) -> Divide1/1
  pfaref/1(pfaref) -> Tan/1
  OR/1 -> [Vdip]  "Voltage_dip"
  Saturation/1 -> Sum4/1  "Iq_inj"
  Qref/1 -> Multiport Switch/2
  Compare To Constant/1 -> OR/1
  [Vt_filt] -> Saturation for Divide by Zeo2/1
  Bus Selector1/1 -> Multiport Switch1/1  "<VFlag>"
  [Iq_cmd] -> Q Priority/1(Iqcmd)
  Q Priority/1(Ipmax) -> Switch1/3
  Gain/1 -> Saturation/1  "Iqv"
  Switch1/1 -> Q Current Saturation1/1
  Sum1/1 -> Voltage Controller/1
  Constant3/1 -> Q Current Saturation1/3
  Switch/1 -> Unary Minus/1, Q Current Saturation/1, [Iqmax]
  Compare To Constant1/1 -> OR/2
  Active Power Filter/1(y) -> Product/2
  P Priority/1(Iqmax) -> Switch/1
  Constant9/1 -> Switch/3
  Q Current Saturation1/1 -> Ip_cmd/1, [Ip_cmd]
  [Vdip] -> Reference Power Filter/2(Vflag)
  [Vdip] -> Current Filter/2(Vflag)
  [Vdip] -> Current Controller/4(Vdip)
  Unary Minus1/1 -> Current Controller/3(umin)
  Mode/1 -> Bus Selector/1
  Bus Selector/1 -> Multiport Switch/1  "<PfFlag>"
  Mode1/1 -> Bus Selector1/1
  Mode2/1 -> Bus Selector2/1
  Mode3/1 -> Bus Selector3/1
  Bus Selector3/1 -> Switch/2  "<PqFlag>"
  Mode4/1 -> Bus Selector4/1

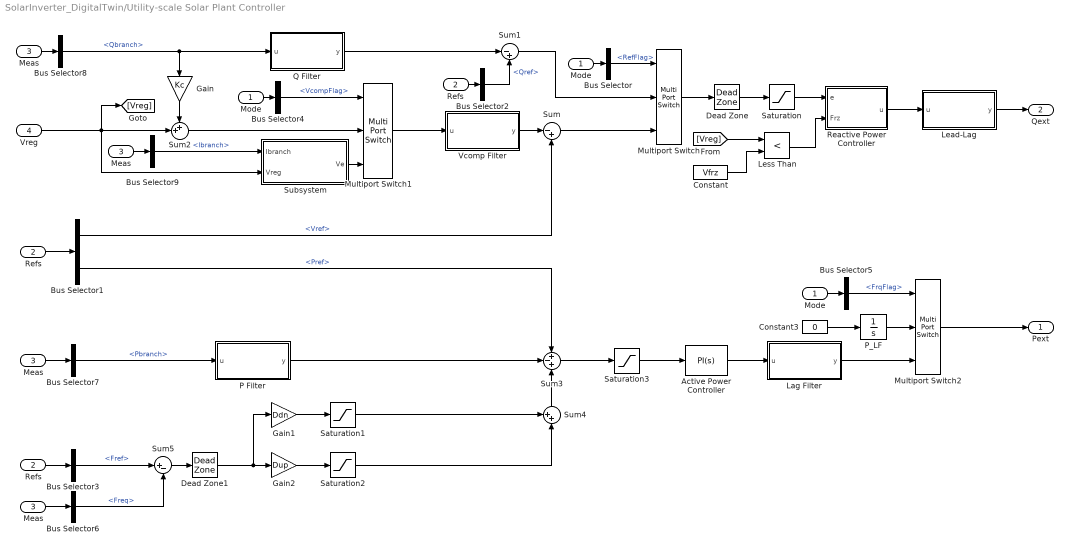
== system SolarInverter_DigitalTwin/Utility-scale Solar Plant Controller ==
  Mode : Inport
  Refs : Inport  Port=2
  " Meas" : Inport  Port=3
  Vreg : Inport  Port=4
  "  Meas" : InportShadow  Port=3
  "  Meas " : InportShadow  Port=3
  " Meas " : InportShadow  Port=3
  " Mode" : InportShadow
  " Refs" : InportShadow  Port=2
  Active Power Controller : simulink/Continuous/PID Controller  Controller=PI  Form=Parallel  TimeDomain=Continuous-time  SampleTime=-1  IntegratorMethod=Forward Euler  FilterMethod=Forward Euler  ControllerParametersSource=internal  P=Kpg  I=Kig  D=0  UseFilter=on  N=100  TunerSelectOption=Transfer Function Based (PID Tuner App)  InitialConditionSource=internal  InitialConditionForIntegrator=1  InitialConditionForFilter=0  DifferentiatorICPrevScaledInput=0  ExternalReset=none  TrackingMode=off  Kt=1  LimitOutput=on  UpperSaturationLimit=Pmax  LowerSaturationLimit=Pmin  LinearizeAsGain=on  AntiWindupMode=none  Kb=1  POutMin=[]  POutMax=[]  IOutMin=[]  IOutMax=[]  DOutMin=[]  DOutMax=[]  NOutMin=[]  NOutMax=[]  SumOutMin=[]  SumOutMax=[]  SaturationOutMin=[]  SaturationOutMax=[]  PParamMin=[]  PParamMax=[]  IParamMin=[]  IParamMax=[]  DParamMin=[]  DParamMax=[]  NParamMin=[]  NParamMax=[]  KbParamMin=[]  KbParamMax=[]  KtParamMin=[]  KtParamMax=[]  KbOutMin=[]  KbOutMax=[]  KtOutMin=[]  KtOutMax=[]  IntegratorOutMin=[]  IntegratorOutMax=[]  FilterOutMin=[]  FilterOutMax=[]  SumI1OutMin=[]  SumI1OutMax=[]  SumI2OutMin=[]  SumI2OutMax=[]  SumI3OutMin=[]  SumI3OutMax=[]  SumI4OutMin=[]  SumI4OutMax=[]  SumDOutMin=[]  SumDOutMax=[]  DifferentiatorOutMin=[]  DifferentiatorOutMax=[]  FilterDiffOutCoefMin=[]  FilterDiffOutCoefMax=[]  ReciprocalOutMin=[]  ReciprocalOutMax=[]  SumDenOutMin=[]  SumDenOutMax=[]  SumNumOutMin=[]  SumNumOutMax=[]  DivideOutMin=[]  DivideOutMax=[]  IntegratorContinuousStateAttributes=''  IntegratorStateMustResolveToSignalObject=off  IntegratorRTWStateStorageClass=Auto  FilterContinuousStateAttributes=''  FilterStateMustResolveToSignalObject=off  FilterRTWStateStorageClass=Auto  ParallelPVariant=InternalParameters  IdealPVariant=Disabled  IVariant=InternalParameters  DVariant=Disabled  IntegratorVariant=Continuous  SatVariant=Enabled  AWVariant=Passthrough  PCopyVariant=Disabled  TRVariant=Disabled  FdbkBlocksVariant=Forward  IdealPFdbkVariant=Disabled  SatFdbkVariant=Disabled  DerivativeFilterVariant=Disabled  NVariant=Disabled  NCopyVariant=Disabled_SignalSpec  FilterICVariant=Disabled  IntegratorICVariant=InternalICs  ExternalResetVariant=Disabled  TRSumVariant=Passthrough  SumFdbkVariant=Disabled  SumVariant=Sum_PI
  Bus Selector : BusSelector  OutputSignals=RefFlag
  Bus Selector1 : BusSelector  OutputSignals=Vref,Pref
  Bus Selector2 : BusSelector  OutputSignals=Qref
  Bus Selector3 : BusSelector  OutputSignals=Fref
  Bus Selector4 : BusSelector  OutputSignals=VcompFlag
  Bus Selector5 : BusSelector  OutputSignals=FrqFlag
  Bus Selector6 : BusSelector  OutputSignals=Freq
  Bus Selector7 : BusSelector  OutputSignals=Pbranch
  Bus Selector8 : BusSelector  OutputSignals=Qbranch
  Bus Selector9 : BusSelector  OutputSignals=Ibranch
  Constant : Constant  Value=Vfrz
  Constant3 : Constant  Value=0
  Dead Zone : DeadZone  LowerValue=-db1  UpperValue=db1  SaturateOnIntegerOverflow=on
  Dead Zone1 : DeadZone  LowerValue=fdbd1  UpperValue=fdbd2  SaturateOnIntegerOverflow=on
  Gain : Gain  Gain=Kc
  Gain1 : Gain  Gain=Ddn
  Gain2 : Gain  Gain=Dup
  Lag Filter : Subsystem  mask{k=1, tau=Tlag, vmax=Inf, vmin=-Inf}
      mask Display: fprintf('1\n------------\n(1 + s Tlag)');
  Lead-Lag : Subsystem  mask{ta=Tft, tb=Tfv}
      mask prompts: ta "numerator tau (ta)"; tb "denominator tau  (tb)"
      mask Display: fprintf('(1 + s Tft)\n------------\n(1 + s Tfv)');
  Less Than : RelationalOperator  Operator=<  OutDataTypeStr=boolean  RndMeth=Simplest
  "Mode " : InportShadow
  Multiport Switch : MultiPortSwitch  DataPortOrder=Zero-based contiguous  Inputs=2  zeroidx=on
  Multiport Switch1 : MultiPortSwitch  DataPortOrder=Zero-based contiguous  Inputs=2  zeroidx=on
  Multiport Switch2 : MultiPortSwitch  DataPortOrder=Zero-based contiguous  Inputs=2  zeroidx=on
  P Filter : Subsystem  mask{k=1, tau=Tp, vmax=Inf, vmin=-Inf}
      mask Display: fprintf('1\n------------\n(1 + s Tfltr)');
  P_LF : Integrator  InitialCondition=1
  Q Filter : Subsystem  mask{k=1, tau=Tfltr, vmax=Inf, vmin=-Inf}
      mask Display: fprintf('1\n------------\n(1 + s Tfltr)');
  Reactive Power Controller : Subsystem
  "Refs " : InportShadow  Port=2
  Saturation : Saturate  UpperLimit=emax  LowerLimit=emin
  Saturation1 : Saturate  UpperLimit=0  LowerLimit=-inf
  Saturation2 : Saturate  UpperLimit=inf  LowerLimit=0
  Saturation3 : Saturate  UpperLimit=femax  LowerLimit=femin
  Subsystem : Subsystem
  Sum : Sum  Inputs=|-+
  Sum1 : Sum  Inputs=|-+
  Sum2 : Sum  Inputs=++|
  Sum3 : Sum  Inputs=+-+
  Sum4 : Sum  Inputs=++|
  Sum5 : Sum  Inputs=|+-
  Vcomp Filter : Subsystem  mask{k=1, tau=Tfltr, vmax=Inf, vmin=-Inf}
      mask Display: fprintf('1\n------------\n(1 + s Tfltr)');
  Pext : Outport  VectorParamsAs1DForOutWhenUnconnected=off
  Qext : Outport  Port=2  VectorParamsAs1DForOutWhenUnconnected=off
  wires:
  Vreg/1 -> [Vreg], Sum2/2, Subsystem/2(Vreg)
  "  Meas "/1 -> Bus Selector9/1
  "  Meas"/1 -> Bus Selector8/1
  " Meas "/1 -> Bus Selector7/1
  " Meas"/1 -> Bus Selector6/1
  " Mode"/1 -> Bus Selector5/1
  Bus Selector4/1 -> Multiport Switch1/1  "<VcompFlag>"
  "Mode "/1 -> Bus Selector4/1
  " Refs"/1 -> Bus Selector3/1
  "Refs "/1 -> Bus Selector2/1
  Refs/1 -> Bus Selector1/1
  Mode/1 -> Bus Selector/1
  Bus Selector1/1 -> Sum/2  "<Vref>"
  Gain/1 -> Sum2/1
  P Filter/1(y) -> Sum3/2
  Bus Selector6/1 -> Sum5/2  "<Freq>"
  Bus Selector8/1 -> Q Filter/1(u), Gain/1  "<Qbranch>"
  Bus Selector3/1 -> Sum5/1  "<Fref>"
  Multiport Switch1/1 -> Vcomp Filter/1(u)
  Sum2/1 -> Multiport Switch1/2
  Vcomp Filter/1(y) -> Sum/1
  Reactive Power Controller/1(u) -> Lead-Lag/1(u)
  Bus Selector2/1 -> Sum1/2  "<Qref>"
  Lead-Lag/1(y) -> Qext/1
  Subsystem/1(Ve) -> Multiport Switch1/3
  Bus Selector1/2 -> Sum3/1  "<Pref>"
  Bus Selector7/1 -> P Filter/1(u)  "<Pbranch>"
  Gain2/1 -> Saturation2/1
  Saturation2/1 -> Sum4/2
  Active Power Controller/1 -> Lag Filter/1(u)
  Lag Filter/1(y) -> Multiport Switch2/3
  Bus Selector5/1 -> Multiport Switch2/1  "<FrqFlag>"
  Dead Zone1/1 -> Gain2/1, Gain1/1
  Multiport Switch2/1 -> Pext/1
  Multiport Switch/1 -> Dead Zone/1
  Gain1/1 -> Saturation1/1
  Sum3/1 -> Saturation3/1
  Bus Selector9/1 -> Subsystem/1(Ibranch)  "<Ibranch>"
  Bus Selector/1 -> Multiport Switch/1  "<RefFlag>"
  Saturation/1 -> Reactive Power Controller/1(e)
  Sum5/1 -> Dead Zone1/1
  Saturation1/1 -> Sum4/1
  Sum1/1 -> Multiport Switch/2
  Sum4/1 -> Sum3/3
  Q Filter/1(y) -> Sum1/1
  Saturation3/1 -> Active Power Controller/1
  Dead Zone/1 -> Saturation/1
  Constant3/1 -> P_LF/1
  Sum/1 -> Multiport Switch/3
  [Vreg] -> Less Than/1
  Less Than/1 -> Reactive Power Controller/2(Frz)
  Constant/1 -> Less Than/2
  P_LF/1 -> Multiport Switch2/2

== system SolarInverter_DigitalTwin/Renewable Grid-Connection/Break F Loop ==
  u : Inport
  Gain2 : Gain  Gain=1/tau
  Integrator2 : Integrator  InitialCondition=1
  Sum3 : Sum  Inputs=|+-
  to PU1 : Gain  Gain=toPU
  to PU7 : Gain  Gain=1/toPU
  y : Outport  VectorParamsAs1DForOutWhenUnconnected=off
  wires:
  to PU1/1 -> y/1
  to PU7/1 -> Sum3/1
  u/1 -> to PU7/1
  Sum3/1 -> Gain2/1
  Integrator2/1 -> Sum3/2, to PU1/1
  Gain2/1 -> Integrator2/1

== system SolarInverter_DigitalTwin/Renewable Grid-Connection/Break P Loop ==
  u : Inport
  Gain2 : Gain  Gain=1/tau
  Integrator2 : Integrator  InitialCondition=1
  Sum3 : Sum  Inputs=|+-
  to PU1 : Gain  Gain=toPU
  to PU7 : Gain  Gain=1/toPU
  y : Outport  VectorParamsAs1DForOutWhenUnconnected=off
  wires:
  Gain2/1 -> Integrator2/1
  Integrator2/1 -> to PU1/1, Sum3/2
  Sum3/1 -> Gain2/1
  u/1 -> to PU7/1
  to PU7/1 -> Sum3/1
  to PU1/1 -> y/1

== system SolarInverter_DigitalTwin/Renewable Grid-Connection/Break Q Loop ==
  u : Inport
  Gain2 : Gain  Gain=1/tau
  Integrator2 : Integrator
  Sum3 : Sum  Inputs=|+-
  to PU1 : Gain  Gain=toPU
  to PU7 : Gain  Gain=1/toPU
  y : Outport  VectorParamsAs1DForOutWhenUnconnected=off
  wires:
  to PU1/1 -> y/1
  to PU7/1 -> Sum3/1
  u/1 -> to PU7/1
  Sum3/1 -> Gain2/1
  Integrator2/1 -> Sum3/2, to PU1/1
  Gain2/1 -> Integrator2/1

== system SolarInverter_DigitalTwin/Renewable Grid-Connection/Break V Loop ==
  u : Inport
  Gain2 : Gain  Gain=1/tau
  Integrator2 : Integrator  InitialCondition=1
  Sum3 : Sum  Inputs=|+-
  to PU1 : Gain  Gain=toPU
  to PU7 : Gain  Gain=1/toPU
  y : Outport  VectorParamsAs1DForOutWhenUnconnected=off
  wires:
  Gain2/1 -> Integrator2/1
  Integrator2/1 -> to PU1/1, Sum3/2
  Sum3/1 -> Gain2/1
  u/1 -> to PU7/1
  to PU7/1 -> Sum3/1
  to PU1/1 -> y/1

== system SolarInverter_DigitalTwin/Renewable Grid-Connection/Clamping Integrator ==
  LVMax : Inport
  e : Inport  Port=2
  Constant : Constant  Value=-inf
  Constant1 : Constant  Value=0
  Integrator1 : Integrator  InitialCondition=1
  Saturation Dynamic : simulink/Discontinuities/Saturation Dynamic  OutMin=[]  OutMax=[]  OutDataTypeStr=Inherit: Same as second input  OutDataType=fixdt(1, 16)  OutScaling=2^-10  DoSatur=off
  Subsystem : Subsystem
  Switch1 : Switch  Criteria=u2 > Threshold
  u : Outport  VectorParamsAs1DForOutWhenUnconnected=off
  wires:
  Saturation Dynamic/1 -> u/1  "u"
  Subsystem/1(Clamp) -> Switch1/2
  Constant/1 -> Saturation Dynamic/3
  Switch1/1 -> Integrator1/1
  LVMax/1 -> Subsystem/3(ymax), Saturation Dynamic/1
  Integrator1/1 -> Subsystem/2(preSat), Saturation Dynamic/2
  e/1 -> Subsystem/1(preIntegrator), Switch1/3
  Constant1/1 -> Switch1/1

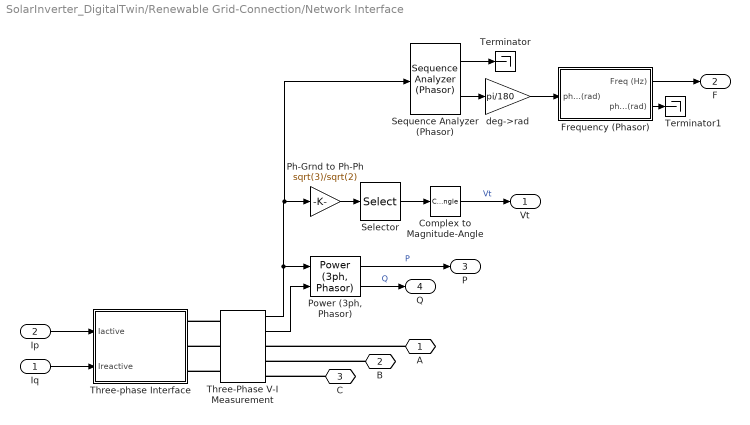
== system SolarInverter_DigitalTwin/Renewable Grid-Connection/Network Interface ==
  Iq : Inport
  Ip : Inport  Port=2
  Complex to Magnitude-Angle : ComplexToMagnitudeAngle  Output=Magnitude
  Frequency (Phasor) : Subsystem  DialogController=POWERSYS.PowerSysDialog  LoadFcn=sps_rtmsupport('LoadFcn', gcbh);  StartFcn=sps_rtmsupport('StartFcn', gcbh);  StopFcn=sps_rtmsupport('StopFcn', gcbh);  mask(Frequency (Phasor)){Fn=Fnom, T=0.01}
      mask prompts: Fn "Nominal frequency (Hz):"; T "Time constant T for derivative (s):"
      mask help:
      | Frequency is computed by derivative of input phase angle variation with respect to a synchronous phasor rotating at nominal frequency, using the following transfer function:
      |
      |      Hd = s / (1+T.s)
      |
      | The unwraped phase angle (without 2*pi discontinuities) is available at output 2.
      settings: CopyFcn=sps_rtmsupport('CopyFcn', gcbh);  DeleteFcn=sps_rtmsupport('DeleteFcn', gcbh);  UndoDeleteFcn=sps_rtmsupport('UndoDeleteFcn', gcbh);  ModelCloseFcn=sps_rtmsupport('ModelCloseFcn', gcbh);  PreSaveFcn=sps_rtmsupport('PreSaveFcn', gcbh);  PostSaveFcn=sps_rtmsupport('PostSaveFcn', gcbh);  NameChangeFcn=sps_rtmsupport('NameChangeFcn', gcbh);  PreCopyFcn=sps_rtmsupport('PreCopyFcn', gcbh);  OpenFcn=sps_rtmsupport('OpenFcn', gcbh, []);  CloseFcn=sps_rtmsupport('CloseFcn', gcbh);  PreDeleteFcn=sps_rtmsupport('PreDeleteFcn', gcbh);
      mask Help: helpview(psbhelp);
      mask Display:
      | port_label('input',1,'Phase (rad)')
      | port_label('output',1,'Freq (Hz)')
      | port_label('output',2,'\DeltaPhi (rad)', 'texmode', 'on')
  Ph-Grnd to Ph-Ph : Gain  Gain=sqrt(3)/sqrt(2)
  "Power (3ph, Phasor)" : powerlib_meascontrol/Measurements/Power (3ph, Phasor)
      settings: SourceProductName=Simscape Electrical  SourceProductBaseCode=PS
  Selector : Selector  InputPortWidth=3  IndexOptions=Index vector (dialog)  Indices=[1]  OutputSizes=1
  Sequence Analyzer (Phasor) : powerlib_meascontrol/Measurements/Sequence Analyzer (Phasor)  seq=Positive
      settings: SourceProductName=Simscape Electrical  SourceProductBaseCode=PS
  Terminator : Terminator
  Terminator1 : Terminator
  Three-Phase V-I Measurement : powerlib/Measurements/Three-Phase V-I Measurement  VoltageMeasurement=phase-to-ground  SetLabelV=off  LabelV=Vabc  Vpu=off  VpuLL=on  CurrentMeasurement=yes  SetLabelI=off  LabelI=Iabc  Ipu=off  Pbase=Pnom  Vbase=Vnom  OutputType=Complex  PhasorSimulation=on  PSBequivalent=0
      settings: SourceProductName=Simscape Electrical
  Three-phase Interface : Subsystem
  deg->rad : Gain  Gain=pi/180
  A : PMIOPort  Side=Right
  B : PMIOPort  Port=2  Side=Right
  C : PMIOPort  Port=3  Side=Right
  Vt : Outport  VectorParamsAs1DForOutWhenUnconnected=off
  F : Outport  Port=2  VectorParamsAs1DForOutWhenUnconnected=off
  P : Outport  Port=3  VectorParamsAs1DForOutWhenUnconnected=off
  Q : Outport  Port=4  VectorParamsAs1DForOutWhenUnconnected=off
  wires:
  Three-Phase V-I Measurement/1 -> "Power (3ph, Phasor)"/1, Sequence Analyzer (Phasor)/1, Ph-Grnd to Ph-Ph/1
  Three-Phase V-I Measurement/2 -> "Power (3ph, Phasor)"/2
  Selector/1 -> Complex to Magnitude-Angle/1
  Iq/1 -> Three-phase Interface/2(Ireactive)
  Ph-Grnd to Ph-Ph/1 -> Selector/1
  Complex to Magnitude-Angle/1 -> Vt/1  "Vt"
  "Power (3ph, Phasor)"/1 -> P/1  "P"
  Ip/1 -> Three-phase Interface/1(Iactive)
  "Power (3ph, Phasor)"/2 -> Q/1  "Q"
  Sequence Analyzer (Phasor)/2 -> deg->rad/1
  Sequence Analyzer (Phasor)/1 -> Terminator/1
  deg->rad/1 -> Frequency (Phasor)/1(phase (rad))
  Frequency (Phasor)/1(Freq (Hz)) -> F/1
  Frequency (Phasor)/2("phase (rad) ") -> Terminator1/1
  connections:
  Three-Phase V-I Measurement/LConn3 -- Three-phase Interface/RConn3
  B/RConn1 -- Three-Phase V-I Measurement/RConn2
  Three-Phase V-I Measurement/LConn1 -- Three-phase Interface/RConn1
  A/RConn1 -- Three-Phase V-I Measurement/RConn1
  C/RConn1 -- Three-Phase V-I Measurement/RConn3
  Three-Phase V-I Measurement/LConn2 -- Three-phase Interface/RConn2

== system SolarInverter_DigitalTwin/Renewable Grid-Connection/Q Current Filter ==
  u : Inport
  1/(taus+1) : Subsystem  mask{tau=tau, vmax=vmax, vmin=vmin}
      mask prompts: tau "Time Constant"
  k : Gain  Gain=k
  y : Outport  VectorParamsAs1DForOutWhenUnconnected=off
  wires:
  1/(taus+1)/1(y) -> y/1
  u/1 -> k/1
  k/1 -> 1/(taus+1)/1(u)

== system SolarInverter_DigitalTwin/Renewable Grid-Connection/Voltage Filter ==
  u : Inport
  1/(taus+1) : Subsystem  mask{tau=tau, vmax=vmax, vmin=vmin}
      mask prompts: tau "Time Constant"
  k : Gain  Gain=k
  y : Outport  VectorParamsAs1DForOutWhenUnconnected=off
  wires:
  k/1 -> 1/(taus+1)/1(u)
  u/1 -> k/1
  1/(taus+1)/1(y) -> y/1

== system SolarInverter_DigitalTwin/Utility-scale Solar Electrical Controller/Active Power Filter ==
  u : Inport
  1/(taus+1) : Subsystem  mask{tau=tau, vmax=vmax, vmin=vmin}
      mask prompts: tau "Time Constant"
  k : Gain  Gain=k
  y : Outport  VectorParamsAs1DForOutWhenUnconnected=off
  wires:
  k/1 -> 1/(taus+1)/1(u)
  u/1 -> k/1
  1/(taus+1)/1(y) -> y/1

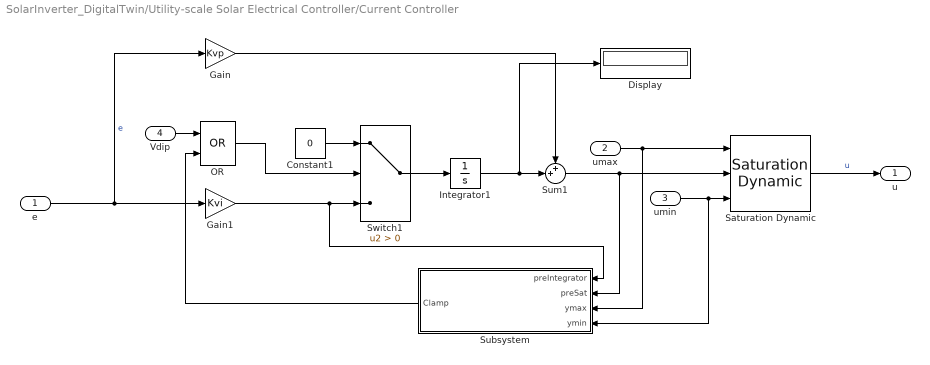
== system SolarInverter_DigitalTwin/Utility-scale Solar Electrical Controller/Current Controller ==
  e : Inport
  umax : Inport  Port=2
  umin : Inport  Port=3
  Vdip : Inport  Port=4
  Constant1 : Constant  Value=0
  Display : Display
  Gain : Gain  Gain=Kvp
  Gain1 : Gain  Gain=Kvi
  Integrator1 : Integrator
  OR : Logic  Operator=OR  AllPortsSameDT=off  OutDataTypeStr=boolean
  Saturation Dynamic : simulink/Discontinuities/Saturation Dynamic  OutMin=[]  OutMax=[]  OutDataTypeStr=Inherit: Same as second input  OutDataType=fixdt(1, 16)  OutScaling=2^-10  DoSatur=off
  Subsystem : Subsystem
  Sum1 : Sum  Inputs=++|
  Switch1 : Switch  Criteria=u2 > Threshold
  u : Outport  VectorParamsAs1DForOutWhenUnconnected=off
  wires:
  Gain/1 -> Sum1/1
  e/1 -> Gain/1, Gain1/1  "e"
  Constant1/1 -> Switch1/1
  umax/1 -> Subsystem/3(ymax), Saturation Dynamic/1
  Integrator1/1 -> Display/1, Sum1/2
  Gain1/1 -> Subsystem/1(preIntegrator), Switch1/3
  Switch1/1 -> Integrator1/1
  Saturation Dynamic/1 -> u/1  "u"
  Sum1/1 -> Subsystem/2(preSat), Saturation Dynamic/2
  umin/1 -> Subsystem/4(ymin), Saturation Dynamic/3
  Vdip/1 -> OR/1
  Subsystem/1(Clamp) -> OR/2
  OR/1 -> Switch1/2

== system SolarInverter_DigitalTwin/Utility-scale Solar Electrical Controller/Current Filter ==
  u : Inport
  Vflag : Inport  Port=2
  1/(taus+1) : Subsystem  mask{tau=tau, vmax=vmax, vmin=vmin}
      mask prompts: tau "Time Constant"
  k : Gain  Gain=k
  y : Outport  VectorParamsAs1DForOutWhenUnconnected=off
  wires:
  1/(taus+1)/1(y) -> y/1
  u/1 -> k/1
  k/1 -> 1/(taus+1)/1(u)
  Vflag/1 -> 1/(taus+1)/2(Vflag)

== system SolarInverter_DigitalTwin/Utility-scale Solar Electrical Controller/P Priority ==
  Ipcmd : Inport
  Constant8 : Constant  Value=Imax
  Sqrt : Sqrt  SaturateOnIntegerOverflow=on
  Square : Math  Operator=square  SaturateOnIntegerOverflow=on
  Square1 : Math  Operator=square  SaturateOnIntegerOverflow=on
  Sum2 : Sum  Inputs=|+-
  Iqmax : Outport  VectorParamsAs1DForOutWhenUnconnected=off
  wires:
  Sqrt/1 -> Iqmax/1
  Sum2/1 -> Sqrt/1
  Constant8/1 -> Square/1
  Square1/1 -> Sum2/2
  Square/1 -> Sum2/1
  Ipcmd/1 -> Square1/1

== system SolarInverter_DigitalTwin/Utility-scale Solar Electrical Controller/Q Priority ==
  Iqcmd : Inport
  Constant8 : Constant  Value=Imax
  Sqrt : Sqrt  SaturateOnIntegerOverflow=on
  Square : Math  Operator=square  SaturateOnIntegerOverflow=on
  Square1 : Math  Operator=square  SaturateOnIntegerOverflow=on
  Sum2 : Sum  Inputs=|+-
  Ipmax : Outport  VectorParamsAs1DForOutWhenUnconnected=off
  wires:
  Sqrt/1 -> Ipmax/1
  Sum2/1 -> Sqrt/1
  Constant8/1 -> Square/1
  Square1/1 -> Sum2/2
  Square/1 -> Sum2/1
  Iqcmd/1 -> Square1/1

== system SolarInverter_DigitalTwin/Utility-scale Solar Electrical Controller/Reference Power Filter ==
  u : Inport
  Vflag : Inport  Port=2
  1/(taus+1) : Subsystem  mask{tau=tau, vmax=vmax, vmin=vmin}
      mask prompts: tau "Time Constant"
  k : Gain  Gain=k
  y : Outport  VectorParamsAs1DForOutWhenUnconnected=off
  wires:
  Vflag/1 -> 1/(taus+1)/2(Vflag)
  k/1 -> 1/(taus+1)/1(u)
  u/1 -> k/1
  1/(taus+1)/1(y) -> y/1

== system SolarInverter_DigitalTwin/Utility-scale Solar Electrical Controller/Vref0 ==
  Constant6 : Constant  Value=0
  Init_Val : Integrator  InitialCondition=1
  Vref0 : Outport  VectorParamsAs1DForOutWhenUnconnected=off
  wires:
  Constant6/1 -> Init_Val/1
  Init_Val/1 -> Vref0/1

== system SolarInverter_DigitalTwin/Utility-scale Solar Electrical Controller/Vt Filter ==
  u : Inport
  1/(taus+1) : Subsystem  mask{tau=tau, vmax=vmax, vmin=vmin}
      mask prompts: tau "Time Constant"
  k : Gain  Gain=k
  y : Outport  VectorParamsAs1DForOutWhenUnconnected=off
  wires:
  k/1 -> 1/(taus+1)/1(u)
  u/1 -> k/1
  1/(taus+1)/1(y) -> y/1

== system SolarInverter_DigitalTwin/Utility-scale Solar Electrical Controller/pfaref ==
  Constant6 : Constant  Value=0
  Init_Val : Integrator
  pfaref : Outport  VectorParamsAs1DForOutWhenUnconnected=off
  wires:
  Constant6/1 -> Init_Val/1
  Init_Val/1 -> pfaref/1

== system SolarInverter_DigitalTwin/Utility-scale Solar Plant Controller/Lag Filter ==
  u : Inport
  1/(taus+1) : Subsystem  mask{tau=tau, vmax=vmax, vmin=vmin}
      mask prompts: tau "Time Constant"
  k : Gain  Gain=k
  y : Outport  VectorParamsAs1DForOutWhenUnconnected=off
  wires:
  k/1 -> 1/(taus+1)/1(u)
  u/1 -> k/1
  1/(taus+1)/1(y) -> y/1

== system SolarInverter_DigitalTwin/Utility-scale Solar Plant Controller/Lead-Lag ==
  note: disable integrator and pass through signal if tb is zero
  u : Inport
  Constant : Constant  Value=tb
  Gain : Gain  Gain=1/(tb+eps)
  Gain1 : Gain  Gain=ta
  Integrator : Integrator
  Sum : Sum  Inputs=|+-
  Sum1 : Sum  Inputs=++|
  Switch : Switch  Criteria=u2 > Threshold
  Switch1 : Switch  Criteria=u2 > Threshold
  y : Outport  VectorParamsAs1DForOutWhenUnconnected=off
  wires:
  Sum/1 -> Gain/1
  Gain/1 -> Switch/1, Gain1/1
  Gain1/1 -> Sum1/1
  Integrator/1 -> Sum1/2, Sum/2
  u/1 -> Switch1/3, Sum/1
  Constant/1 -> Switch1/2, Switch/3, Switch/2
  Switch/1 -> Integrator/1
  Sum1/1 -> Switch1/1
  Switch1/1 -> y/1
